simulink model "FDM_Cau3"  (R2017b)
settings: Solver=VariableStepAuto  StartTime=0.0  StopTime=10.0  FixedStep=1e-5  RelTol=1e-3  EnableMultiTasking=on
libraries: commanapbnd3 x10
settings Model: Creator=admin  LastModifiedBy=admin
settings DataIOCC: LimitDataPoints=on  SaveFormat=Array
settings OptimizationCC: LifeSpan=inf
settings DebuggingCC: SFUnexpectedBacktrackingDiag=warning  SFNoUnconditionalDefaultTransitionDiag=warning  SFExecutionAtInitializationDiag=none
settings HardwareCC: ProdBitPerPointer=32  ProdBitPerSizeT=32  ProdBitPerPtrDiffT=32  ProdLargestAtomicFloat=None  ProdIntDivRoundTo=Undefined  ProdEndianess=Unspecified  ProdWordSize=32  ProdHWDeviceType=32-bit Generic
settings ModelReferenceCC: PropagateSignalLabelsOutOfModel=off
settings CodeAppCC: StateflowObjectComments=on
settings GRTTargetCC: TargetLangStandard=C89/C90 (ANSI)  GeneratePreprocessorConditionals=Disable all
settings ConfigComp: CovMetricSettings=dw  CovHtmlReporting=on  CovSaveCumulativeToWorkspaceVar=on  CovSaveSingleToWorkspaceVar=on  CovExternalEMLEnable=off

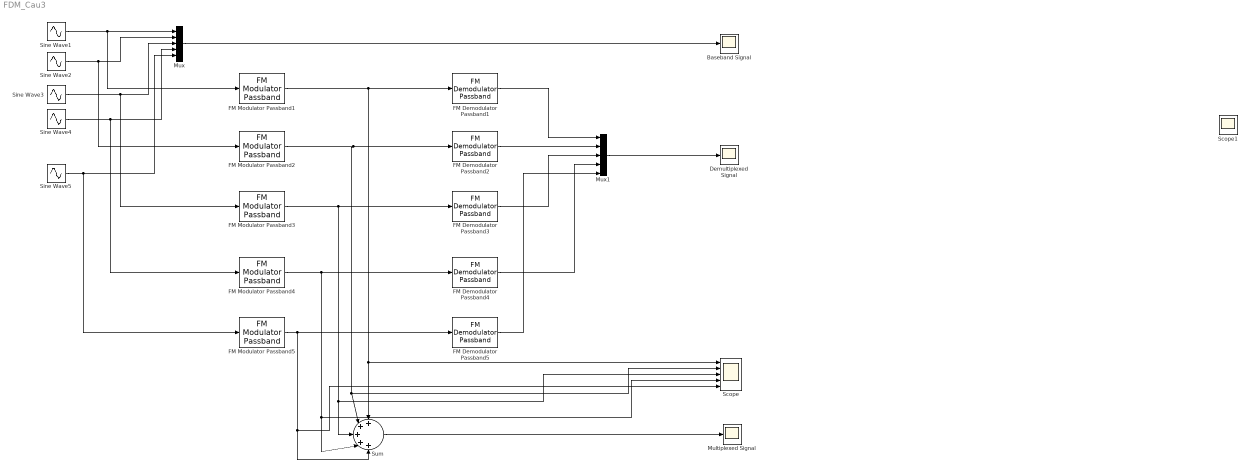
== system FDM_Cau3 ==
  Baseband Signal : Scope
  Demultiplexed Signal : Scope
  FM Demodulator Passband1 : commanapbnd3/FM Demodulator Passband  Fc=11000  Ph=0  Kc=300  Ho=100
      settings: SourceProductName=Communications System Toolbox  SourceProductBaseCode=CM
  FM Demodulator Passband2 : commanapbnd3/FM Demodulator Passband  Fc=12000  Ph=0  Kc=300  Ho=100
      settings: SourceProductName=Communications System Toolbox  SourceProductBaseCode=CM
  FM Demodulator Passband3 : commanapbnd3/FM Demodulator Passband  Fc=13000  Ph=0  Kc=300  Ho=100
      settings: SourceProductName=Communications System Toolbox  SourceProductBaseCode=CM
  FM Demodulator Passband4 : commanapbnd3/FM Demodulator Passband  Fc=14000  Ph=0  Kc=300  Ho=100
      settings: SourceProductName=Communications System Toolbox  SourceProductBaseCode=CM
  FM Demodulator Passband5 : commanapbnd3/FM Demodulator Passband  Fc=14500  Ph=0  Kc=300  Ho=100
      settings: SourceProductName=Communications System Toolbox  SourceProductBaseCode=CM
  FM Modulator Passband1 : commanapbnd3/FM Modulator Passband  Fc=11000  Ph=0  Kc=300
      settings: SourceProductName=Communications System Toolbox  SourceProductBaseCode=CM
  FM Modulator Passband2 : commanapbnd3/FM Modulator Passband  Fc=12000  Ph=0  Kc=300
      settings: SourceProductName=Communications System Toolbox  SourceProductBaseCode=CM
  FM Modulator Passband3 : commanapbnd3/FM Modulator Passband  Fc=13000  Ph=0  Kc=300
      settings: SourceProductName=Communications System Toolbox  SourceProductBaseCode=CM
  FM Modulator Passband4 : commanapbnd3/FM Modulator Passband  Fc=14000  Ph=0  Kc=300
      settings: SourceProductName=Communications System Toolbox  SourceProductBaseCode=CM
  FM Modulator Passband5 : commanapbnd3/FM Modulator Passband  Fc=14500  Ph=0  Kc=300
      settings: SourceProductName=Communications System Toolbox  SourceProductBaseCode=CM
  "Multiplexed Signal " : Scope
  Mux : Mux  Inputs=5
  Mux1 : Mux  Inputs=5
  Scope : Scope  NumInputPorts=5
  Scope1 : Scope
  Sine Wave1 : Sin  Frequency=40*pi  SampleTime=0.0001
  Sine Wave2 : Sin  Frequency=40*pi  Phase=pi/6  SampleTime=0.0001
  Sine Wave3 : Sin  Frequency=40*pi  Phase=-2*pi/6  SampleTime=0.0001
  Sine Wave4 : Sin  Frequency=40*pi  Phase=pi/3  SampleTime=0.0001
  Sine Wave5 : Sin  Frequency=40*pi  Phase=-2*pi/3  SampleTime=0.0001
  Sum : Sum  Inputs=+++++
  wires:
  Sine Wave1/1 -> FM Modulator Passband1/1, Mux/1
  Sine Wave2/1 -> FM Modulator Passband2/1, Mux/2
  Sine Wave3/1 -> FM Modulator Passband3/1, Mux/3
  Sine Wave4/1 -> FM Modulator Passband4/1, Mux/4
  Sine Wave5/1 -> FM Modulator Passband5/1, Mux/5
  Mux/1 -> Baseband Signal/1
  FM Modulator Passband1/1 -> Sum/1, Scope/1, FM Demodulator Passband1/1
  FM Modulator Passband2/1 -> Scope/2, Sum/2, FM Demodulator Passband2/1
  FM Modulator Passband3/1 -> Scope/3, Sum/3, FM Demodulator Passband3/1
  FM Modulator Passband4/1 -> Scope/4, Sum/4, FM Demodulator Passband4/1
  FM Modulator Passband5/1 -> Scope/5, Sum/5, FM Demodulator Passband5/1
  FM Demodulator Passband1/1 -> Mux1/1
  FM Demodulator Passband2/1 -> Mux1/2
  FM Demodulator Passband3/1 -> Mux1/3
  FM Demodulator Passband4/1 -> Mux1/4
  FM Demodulator Passband5/1 -> Mux1/5
  Mux1/1 -> Demultiplexed Signal/1
  Sum/1 -> "Multiplexed Signal "/1
